simulink model "elec_controlled_dcmotor_v1"  (R2013a)
settings: Solver=ode15s  StartTime=0.0  StopTime=10  MaxStep=1  RelTol=1e-3
libraries: fl_lib x5, elec_lib x3, nesl_utility x3
Description:
  | Controlled DC Motor
  | 
  | This model shows how to use the Controlled PWM Voltage and
  | H-Bridge blocks to control a motor. The DC Motor block uses
  | manufacturer datasheet parameters, which specify the motor as
  | delivering 10W mechanical power at 2500 rpm and no-load speed
  | as 4000 rpm when run from a 12V DC supply. Hence if the DC
  | Voltage Source is set to +5V, then the motor should run at 4000
  | rpm. If it is set to +2.5V, then it should run at approximately 2000
  | rpm. The Simulation model parameter is set to Averaged for both
  | the Controlled PWM Voltage and H-Bridge blocks, resulting in fast
  | simulation. To validate the averaged behavior, change the
  | Simulation mode parameter to PWM in both blocks.
  | 
  | 
  | 
  | Copyright 2008-2013 The MathWorks, Inc.
settings Model: Creator=MathWorks  LastModifiedBy=mainster
settings DataIOCC: SignalLoggingSaveFormat=ModelDataLogs
settings OptimizationCC: ExpressionDepthLimit=2147483647  InitFltsAndDblsToZero=on
settings DebuggingCC: SolverPrmCheckMsg=none  FcnCallInpInsideContextMsg=UseLocalSettings  StrictBusMsg=Warning
settings GRTTargetCC: CombineOutputUpdateFcns=off  GRTInterface=on

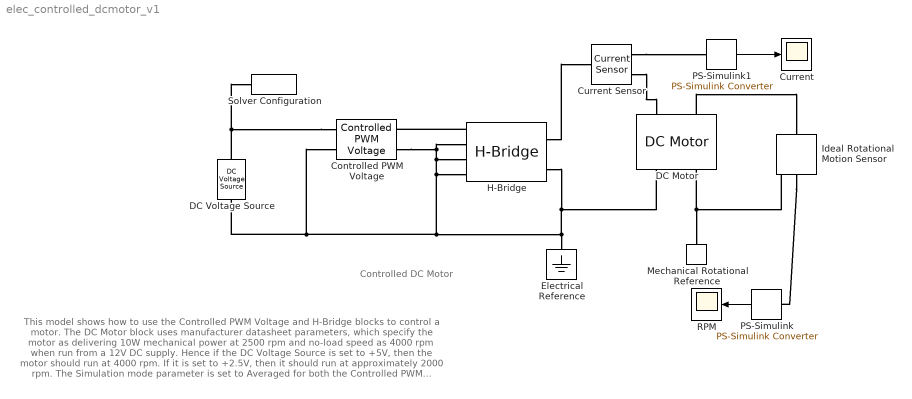
== system elec_controlled_dcmotor_v1 ==
  note: Controlled DC Motor
  note: This model shows how to use the Controlled PWM Voltage and H-Bridge blocks
      | to control a motor. The DC Motor block uses manufacturer datasheet parameters,
      | which specify the motor as delivering 10W mechanical power at 2500 rpm and
      | no-load speed as 4000 rpm when run from a 12V DC supply. Hence if the DC
      | Voltage Source is set to +5V, then the motor should run at 4000 rpm. If it is set
      | to +2.5V, then it should run at approximately 2000 rpm. The Simulation mode
      | parameter is set to Averaged for both the Controlled PWM Voltage and H-Bridge
      | blocks, resulting in fast simulation. To validate the averaged behavior, change the
      | Simulation mode parameter to PWM in both blocks.
  Controlled PWM Voltage : elec_lib/Actuators & Drivers/Drivers/Controlled PWM Voltage  F=4000 Hz  TD=0 s  pulse_width_offset=0 s  Vmin=0 V  Vmax=5 V  Vm=5 V  pwm_or_av=2  event_type=1  sample_time=1e-6 s  LocalVarNames=|current|voltage|power  LocalVarDescs=|Load current (A)|Load voltage (V)|Load power (W)  LocalVarLogging=[0 0 0]
  Current : Scope
      settings: TimeRange=10  YMin=-0.5  YMax=2  SaveName=RPM  SampleTime=0.1
  Current Sensor : fl_lib/Electrical/Electrical Sensors/Current Sensor  i1_Log=off  v1_Log=off  LocalVarNames=|i1|v1  LocalVarDescs=|i1|v1  LocalVarLogging=[]
  DC Voltage Source : fl_lib/Electrical/Electrical Sources/DC Voltage Source  v0=2.5 V  i_Log=off  v_Log=off  LocalVarNames=|current|voltage|power  LocalVarDescs=|Current (A)|Voltage (V)|Power (W)  LocalVarLogging=[0 0 0]
  DC Motor : elec_lib/Actuators & Drivers/Rotational Actuators/DC Motor  parameterization=3  Ra=3.9 Ohm  La=0.01 H  emf_or_torque=1  Kv=7.2e-05 V/rpm  Ki=6.876e-04 N*m/A  T_stall=2.4e-04 N*m  w_max=4000 rpm  w_rated=2500 rpm  P_rated=10 W  V_rated=12 V  J=0.0002 kg*m^2  lam_param=1  lam=1e-06 N*m/(rad/s)  i_noload=0 A  V_i_noload=1.5 V  speed0=0 rpm  current_Log=off  voltage_Log=off  power_Log=off  i2r_Log=off  torque_Log=off  speed_Log=off  LocalVarNames=|current|voltage|power|i2r|torque|speed  LocalVarDescs=|Current (A)|Voltage (V)|Power (W)|Electrical losses (W)|Torque (Nm)|Angular speed (rad/s)  LocalVarLogging=[0 0 0 0 0 0]  alpha=0.00393 1/K  Tmeas=25 C  thermal_mass=100 J/K  initial_temperature=25 C
  Electrical Reference : fl_lib/Electrical/Electrical Elements/Electrical Reference  i_Log=off  LocalVarNames=|i  LocalVarDescs=|i  LocalVarLogging=[]
  H-Bridge : elec_lib/Actuators & Drivers/Drivers/H-Bridge  Venable=2.5 V  Vmax=5 V  Vreverse=2.5 V  Vbrake=2.5 V  Vm=12 V  pwm_or_av=2  discontinuous=0  freewheeling_mode=1  freewheeling_mode_disc=1  Ron=0.1 Ohm  Don=0.1 Ohm  Rload=10 Ohm  Lload=1e-5 H  F=10 kHz  current_Log=off  voltage_Log=off  power_Log=off  LocalVarNames=|current|voltage|power  LocalVarDescs=|Load current (A)|Load voltage (V)|Load power (W)  LocalVarLogging=[0 0 0]
  Ideal Rotational Motion Sensor : fl_lib/Mechanical/Mechanical Sensors/Ideal Rotational Motion Sensor  offset=0 deg  w_Log=off  t_Log=off  phi_Log=off  LocalVarNames=|w|t|phi  LocalVarDescs=|w|t|phi  LocalVarLogging=[]
  Mechanical Rotational Reference : fl_lib/Mechanical/Rotational Elements/Mechanical Rotational Reference  t_Log=off  LocalVarNames=|t  LocalVarDescs=|t  LocalVarLogging=[]
  PS-Simulink : nesl_utility/PS-Simulink Converter  PhysicalDomain=network_engine_domain  SubClassName=ps_output  LeftPortType=input  RightPortType=output  PseudoPeriodic=off  Frequencies=[]  Unit=rpm  AffineConversion=off
  PS-Simulink1 : nesl_utility/PS-Simulink Converter  PhysicalDomain=network_engine_domain  SubClassName=ps_output  LeftPortType=input  RightPortType=output  PseudoPeriodic=off  Frequencies=[]  Unit=A  AffineConversion=off
  RPM : Scope
      settings: YMin=0  YMax=5000  SaveName=RPM1  SampleTime=0.1
  Solver Configuration : nesl_utility/Solver Configuration  PhysicalDomain=network_engine_domain  SubClassName=solver  LeftPortType=input  RightPortType=generic  Accelerate=off  Tones=[]  Harmonics=[]  SimulateNoise=off  Profile=off  UseLocalSampling=off  EnableSwitchedLinearOptims=on  FrequencyDomain=off  UseCCode=off  UseNewInitialization=off  DoDC=off  ResidualTolerance=1e-9  UseLocalSolver=off  LocalSolverChoice=NE_BACKWARD_EULER_ADVANCER  LocalSolverSampleTime=.001  DoFixedCost=off  MaxNonlinIter=3  MaxModeIter=2  LinearAlgebra=Sparse  DelaysMemoryBudget=1024
  wires:
  PS-Simulink/1 -> RPM/1
  PS-Simulink1/1 -> Current/1
  connections:
  DC Motor/LConn2 -- Ideal Rotational Motion Sensor/LConn1
  H-Bridge/LConn1 -- Controlled PWM Voltage/RConn1
  DC Motor/RConn2 -- Mechanical Rotational Reference/LConn1 -- Ideal Rotational Motion Sensor/RConn1
  Ideal Rotational Motion Sensor/RConn2 -- PS-Simulink/LConn1
  Controlled PWM Voltage/LConn1 -- DC Voltage Source/LConn1 -- Solver Configuration/RConn1
  H-Bridge/RConn1 -- Current Sensor/LConn1
  Current Sensor/RConn2 -- DC Motor/LConn1
  Current Sensor/RConn1 -- PS-Simulink1/LConn1
  DC Voltage Source/RConn1 -- Controlled PWM Voltage/LConn2 -- H-Bridge/LConn2 -- Controlled PWM Voltage/RConn2 -- H-Bridge/LConn3 -- H-Bridge/LConn4 -- Electrical Reference/LConn1 -- H-Bridge/RConn2 -- DC Motor/RConn1
